simulink model "Sim2"  (R2017b)
settings: Solver=ode45  StartTime=0.0  StopTime=10  FixedStep=0.001  RelTol=1e-3
undefined symbols (not defined in the file or in its folder): g, psi
settings Model: Creator=Khanh  LastModifiedBy=Khanh

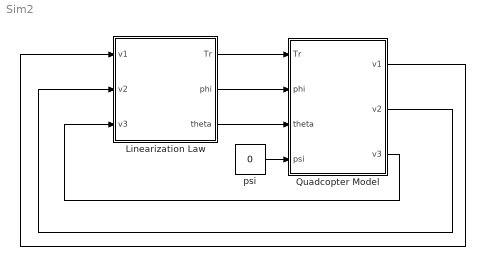
== system Sim2 ==
  Linearization Law : Subsystem
  Quadcopter Model : Subsystem
  psi : Constant  Value=0
  wires:
  psi/1 -> Quadcopter Model/4(psi)
  Linearization Law/3("theta ") -> Quadcopter Model/3(theta)
  Linearization Law/2(phi) -> Quadcopter Model/2(phi)
  Linearization Law/1(Tr) -> Quadcopter Model/1(Tr)
  Quadcopter Model/1(v1) -> Linearization Law/1(v1)
  Quadcopter Model/2(v2) -> Linearization Law/2(v2)
  Quadcopter Model/3(v3) -> Linearization Law/3(v3)

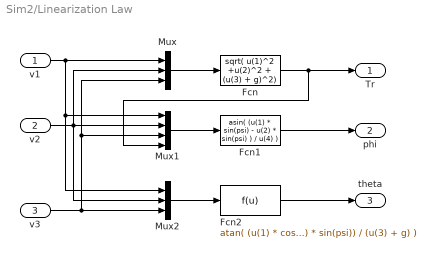
== system Sim2/Linearization Law ==
  v1 : Inport
  v2 : Inport  Port=2
  v3 : Inport  Port=3
  Fcn : Fcn  Expr=sqrt( u(1)^2 +u(2)^2 + (u(3) + g)^2)
  Fcn1 : Fcn  Expr=asin( (u(1) * sin(psi) - u(2) * sin(psi) ) / u(4) )
  Fcn2 : Fcn  Expr=atan( (u(1) * cos(psi) + u(2) * sin(psi)) / (u(3) + g) )
  Mux : Mux  Inputs=3
  Mux1 : Mux
  Mux2 : Mux  Inputs=3
  Tr : Outport
  phi : Outport  Port=2
  "theta " : Outport  Port=3
  wires:
  v1/1 -> Mux/1, Mux2/1, Mux1/1
  v2/1 -> Mux2/2, Mux1/2, Mux/2
  v3/1 -> Mux2/3, Mux1/3, Mux/3
  Fcn/1 -> Mux1/4, Tr/1
  Mux/1 -> Fcn/1
  Fcn1/1 -> phi/1
  Mux1/1 -> Fcn1/1
  Fcn2/1 -> "theta "/1
  Mux2/1 -> Fcn2/1

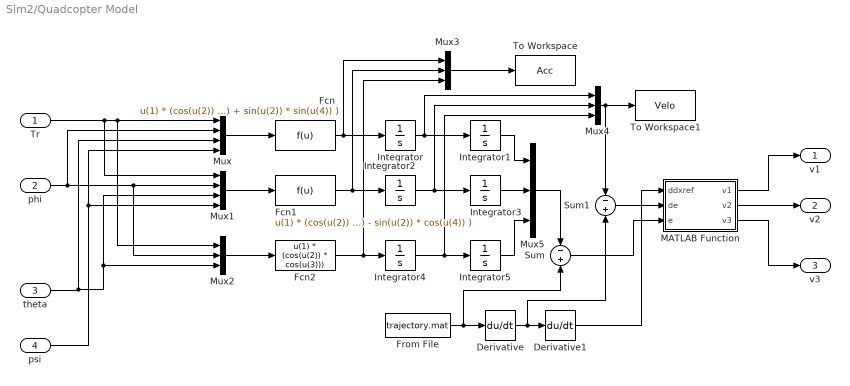
== system Sim2/Quadcopter Model ==
  Tr : Inport
  phi : Inport  Port=2
  theta : Inport  Port=3
  psi : Inport  Port=4
  Derivative : Derivative
  Derivative1 : Derivative
  Fcn : Fcn  Expr=u(1) * (cos(u(2)) * sin(u(3)) * cos(u(4)) + sin(u(2)) * sin(u(4)) )
  Fcn1 : Fcn  Expr=u(1) * (cos(u(2)) * sin(u(3)) * sin(u(4)) - sin(u(2)) * cos(u(4)) )
  Fcn2 : Fcn  Expr=u(1) * (cos(u(2)) * cos(u(3)))
  From File : FromFile  FileName=trajectory.mat  SampleTime=0
  Integrator : Integrator  InitialCondition=5
  Integrator1 : Integrator
  Integrator2 : Integrator  InitialCondition=0.1
  Integrator3 : Integrator
  Integrator4 : Integrator  InitialCondition=0.1
  Integrator5 : Integrator
  MATLAB Function : MATLAB Function  TreatAsAtomicUnit=on
  Mux : Mux
  Mux1 : Mux
  Mux{2..5} (4 alike) : Mux  Inputs=3
  Sum : Sum  Inputs=-+
  Sum1 : Sum  Inputs=-+
  To Workspace : ToWorkspace  VariableName=Acc  SaveFormat=Timeseries  SampleTime=-1
  To Workspace1 : ToWorkspace  VariableName=Velo  SaveFormat=Timeseries  SampleTime=-1
  v1 : Outport
  v2 : Outport  Port=2
  v3 : Outport  Port=3
  wires:
  Mux/1 -> Fcn/1
  Tr/1 -> Mux1/1, Mux2/1, Mux/1
  phi/1 -> Mux2/2, Mux1/2, Mux/2
  theta/1 -> Mux2/3, Mux1/3, Mux/3
  Mux1/1 -> Fcn1/1
  psi/1 -> Mux1/4, Mux/4
  Mux2/1 -> Fcn2/1
  Fcn/1 -> Mux3/1, Integrator/1
  Integrator/1 -> Mux4/1, Integrator1/1
  Fcn1/1 -> Mux3/2, Integrator2/1
  Integrator2/1 -> Mux4/2, Integrator3/1
  Integrator4/1 -> Mux4/3, Integrator5/1
  Fcn2/1 -> Mux3/3, Integrator4/1
  Mux3/1 -> To Workspace/1
  Mux4/1 -> Sum1/1, To Workspace1/1
  MATLAB Function/1(v1) -> v1/1
  MATLAB Function/2(v2) -> v2/1
  MATLAB Function/3(v3) -> v3/1
  Integrator3/1 -> Mux5/2
  Integrator1/1 -> Mux5/1
  Integrator5/1 -> Mux5/3
  From File/1 -> Sum/2, Derivative/1
  Derivative/1 -> Sum1/2, Derivative1/1
  Derivative1/1 -> MATLAB Function/1(ddxref)
  Sum/1 -> MATLAB Function/3(e)
  Mux5/1 -> Sum/1
  Sum1/1 -> MATLAB Function/2(de)

== matlab function Sim2/Quadcopter Model/MATLAB Function ==
  data: ddxref input size=3; v1 output size=1; v2 output size=1; v3 output size=1; de input size=3; e input size=3
function [v1,v2,v3] = fcn(ddxref,de,e)
v1 = ddxref(1) + 4*de(1) * 4*e(1);
v2 = ddxref(2) + 4*de(2) * 4*e(2);
v3 = ddxref(3) + 4*de(3) * 4*e(3);
